simulink model "simulation_UMFCBF"  (R2022a)
settings: Solver=VariableStepAuto  StartTime=0.0  StopTime=simTime  RelTol=1e-3
values from neighbouring files (symbols this model uses):
  a = 0.20    (= 0.2)    [setup_UMFCBF.m]
  Icm = 1/2*m*robot_radius^2    (= 0.225)    [setup_UMFCBF.m]
  Kd = 100    [setup_UMFCBF.m]
  Kp = 2    [setup_UMFCBF.m]
  m = 5    [setup_UMFCBF.m]
  qg = [4 ; -1]    [setup_UMFCBF.m]
  qstart = [-2 0.1 0]'    [setup_UMFCBF.m]
  threshold_skip = 0    [setup_UMFCBF.m]
undefined symbols (not defined in the file or in its folder): clearance, obs, q0, r
libraries: slctrlblks x1
settings Model: Creator=mirkomizzoni  LastModifiedBy=dennis

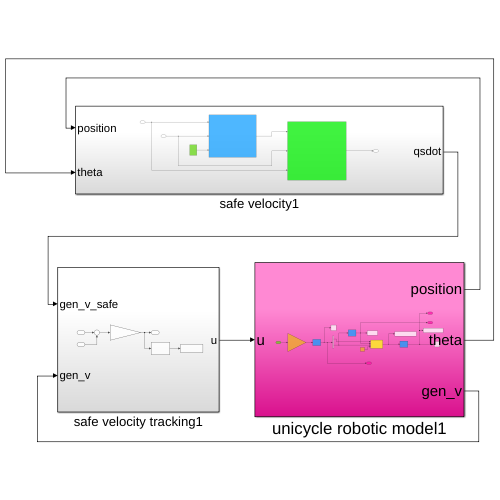
[thumbnail: Simulink's stored preview of the top-level diagram]
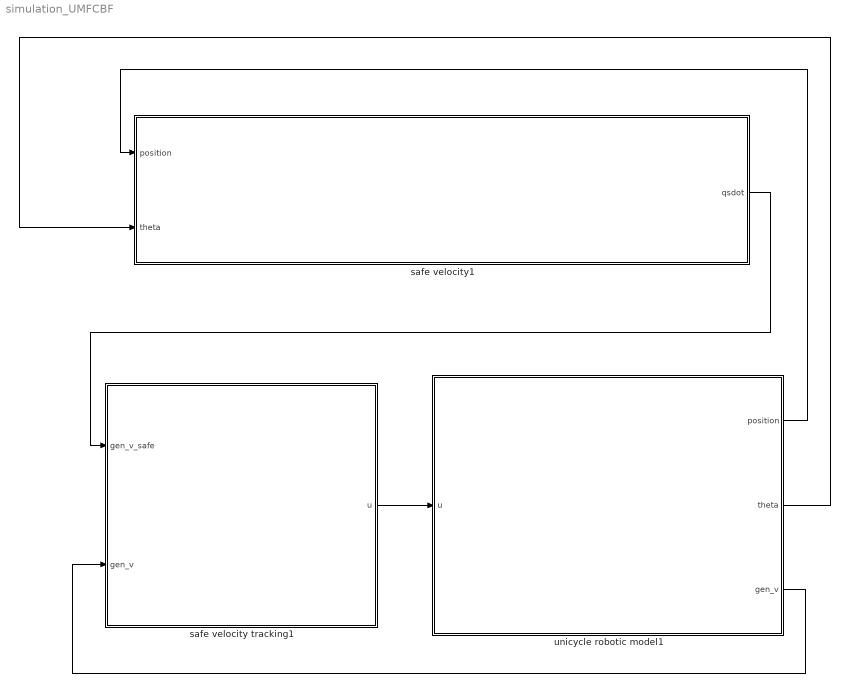
== system simulation_UMFCBF ==
  safe velocity tracking1 : Subsystem
  safe velocity1 : Subsystem
  unicycle robotic model1 : Subsystem
  wires:
  safe velocity1/1(qsdot) -> safe velocity tracking1/1(gen_v_safe)
  safe velocity tracking1/1(u) -> unicycle robotic model1/1(u)
  unicycle robotic model1/3(gen_v) -> safe velocity tracking1/2(gen_v)
  unicycle robotic model1/1(position) -> safe velocity1/1(position)
  unicycle robotic model1/2(theta) -> safe velocity1/2(theta)

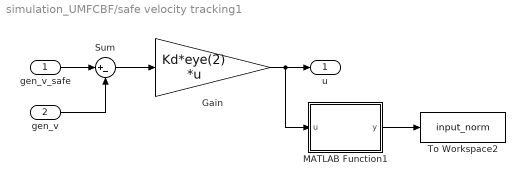
== system simulation_UMFCBF/safe velocity tracking1 ==
  gen_v_safe : Inport
  gen_v : Inport  Port=2
  Gain : Gain  Gain=Kd*eye(2)  Multiplication=Matrix(K*u)
  MATLAB Function1 : MATLAB Function  TreatAsAtomicUnit=on
  Sum : Sum  Inputs=|+-
  To Workspace2 : ToWorkspace  VariableName=input_norm  SaveFormat=Timeseries  SampleTime=0.01
  u : Outport
  wires:
  gen_v/1 -> Sum/2
  gen_v_safe/1 -> Sum/1
  Sum/1 -> Gain/1
  Gain/1 -> u/1, MATLAB Function1/1(u)
  MATLAB Function1/1(y) -> To Workspace2/1

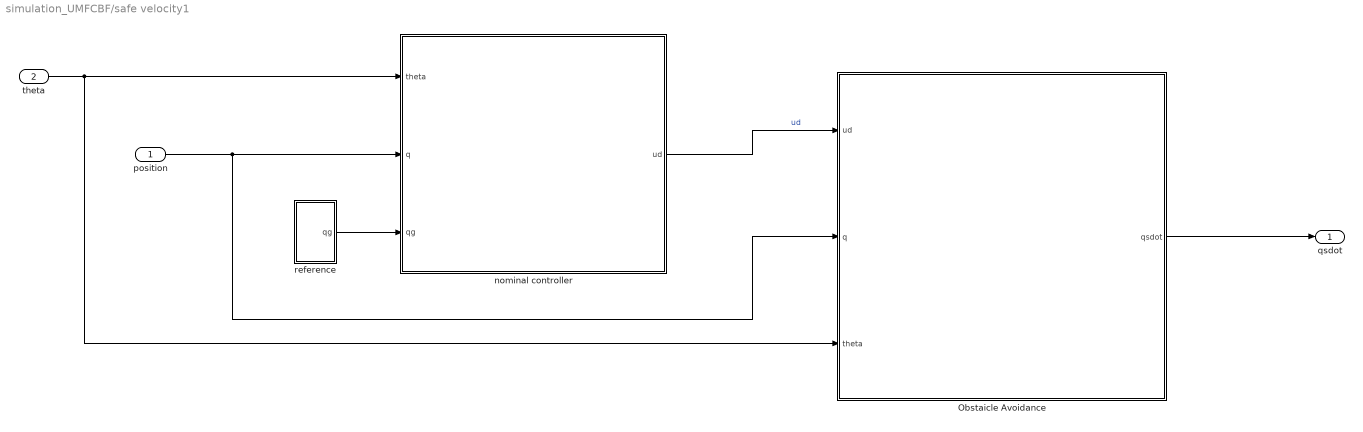
== system simulation_UMFCBF/safe velocity1 ==
  position : Inport
  theta : Inport  Port=2
  Obstaicle Avoidance : Subsystem
  nominal controller : Subsystem
  reference : Subsystem
  qsdot : Outport
  wires:
  reference/1(qg) -> nominal controller/3(qg)
  nominal controller/1(ud) -> Obstaicle Avoidance/1(ud)  "ud"
  Obstaicle Avoidance/1(qsdot) -> qsdot/1
  position/1 -> nominal controller/2(q), Obstaicle Avoidance/2(q)
  theta/1 -> Obstaicle Avoidance/3(theta), nominal controller/1(theta)

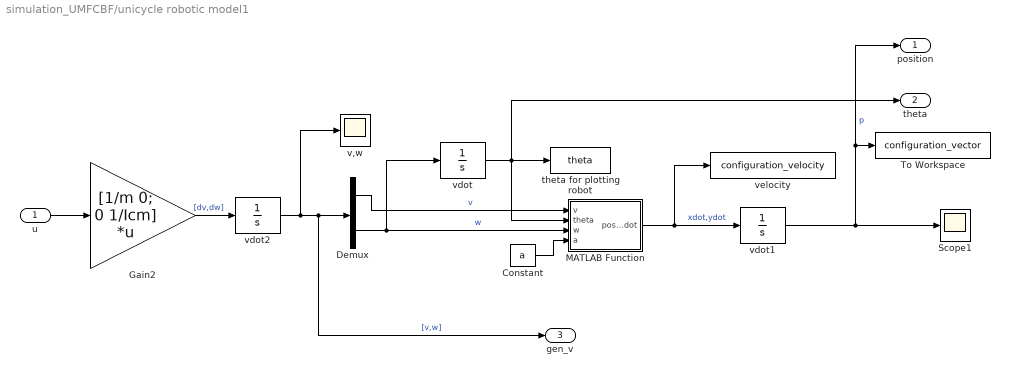
== system simulation_UMFCBF/unicycle robotic model1 ==
  u : Inport
  Constant : Constant  Value=a
  Demux : Demux  Outputs=2
  Gain2 : Gain  Gain=[1/m 0; 0 1/Icm]  Multiplication=Matrix(K*u)
  MATLAB Function : MATLAB Function  TreatAsAtomicUnit=on
  Scope1 : Scope
  To Workspace : ToWorkspace  VariableName=configuration_vector  SaveFormat=Timeseries  SampleTime=0.01
  theta for plotting robot : ToWorkspace  VariableName=theta  SaveFormat=Timeseries  SampleTime=0.01
  v,w : Scope
  vdot : Integrator  InitialCondition=q0(3)
  vdot1 : Integrator  InitialCondition=qstart
  vdot2 : Integrator  InitialCondition=[q0(4); q0(5)]
  velocity : ToWorkspace  VariableName=configuration_velocity  SaveFormat=Timeseries  SampleTime=0.01
  position : Outport
  theta : Outport  Port=2
  gen_v : Outport  Port=3
  wires:
  vdot/1 -> theta/1, theta for plotting robot/1, MATLAB Function/2(theta)
  Demux/2 -> vdot/1, MATLAB Function/3(w)  "w"
  vdot2/1 -> v,w/1, gen_v/1, Demux/1  "[v,w]"
  MATLAB Function/1(positiondot) -> velocity/1, vdot1/1  "xdot,ydot"
  Constant/1 -> MATLAB Function/4(a)
  Gain2/1 -> vdot2/1  "[dv,dw]"
  Demux/1 -> MATLAB Function/1(v)  "v"
  u/1 -> Gain2/1
  vdot1/1 -> position/1, To Workspace/1, Scope1/1  "p"

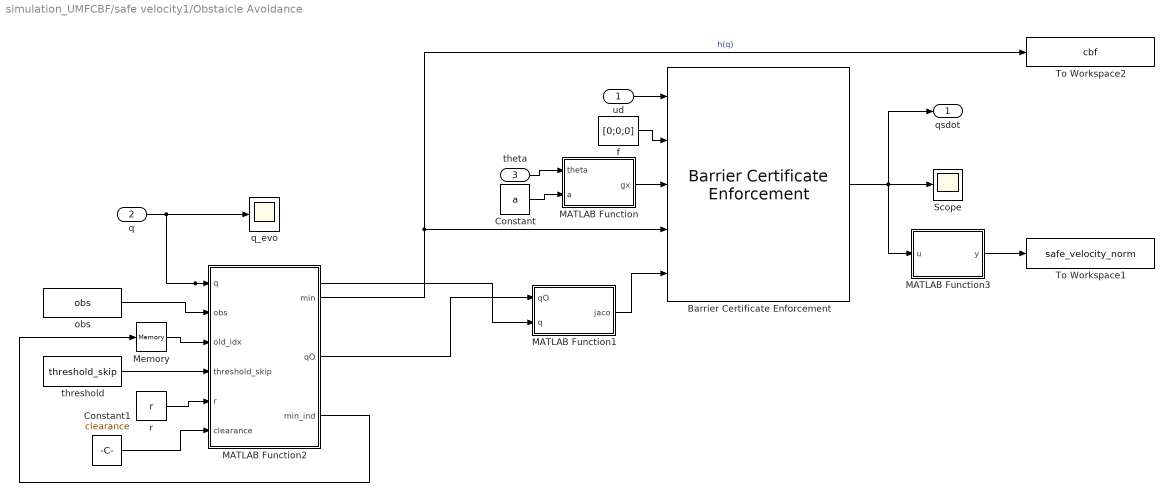
== system simulation_UMFCBF/safe velocity1/Obstaicle Avoidance ==
  ud : Inport
  q : Inport  Port=2
  theta : Inport  Port=3
  Barrier Certificate Enforcement : slctrlblks/Barrier Certificate Enforcement  nx=3  nu=2  nc=1  gamma=alpha  beta=1  external_umax=off  external_umin=off  Ts=0.01  maxiter=200  tol=1e-06  output_exitflag=off
      settings: SourceProductBaseCode=SD
  Constant : Constant  Value=a
  Constant1 : Constant  Value=clearance
  MATLAB Function : MATLAB Function  TreatAsAtomicUnit=on
  MATLAB Function1 : MATLAB Function  TreatAsAtomicUnit=on
  MATLAB Function2 : MATLAB Function  TreatAsAtomicUnit=on
  MATLAB Function3 : MATLAB Function  TreatAsAtomicUnit=on
  Memory : Memory  InitialCondition=1
  Scope : Scope
  To Workspace1 : ToWorkspace  VariableName=safe_velocity_norm  SaveFormat=Timeseries  SampleTime=0.01
  To Workspace2 : ToWorkspace  VariableName=cbf  SaveFormat=Timeseries  SampleTime=0.01
  f : Constant  Value=[0;0;0]  VectorParams1D=off
  obs : Constant  Value=obs  VectorParams1D=off
  q_evo : Scope
  r : Constant  Value=r
  threshold : Constant  Value=threshold_skip  VectorParams1D=off
  qsdot : Outport
  wires:
  MATLAB Function2/2(qO) -> MATLAB Function1/1(qO)
  q/1 -> MATLAB Function2/1(q), MATLAB Function1/2(q), q_evo/1
  MATLAB Function2/3(min_ind) -> Memory/1
  MATLAB Function3/1(y) -> To Workspace1/1
  MATLAB Function2/1(min) -> To Workspace2/1, Barrier Certificate Enforcement/4  "h(q)"
  threshold/1 -> MATLAB Function2/4(threshold_skip)
  f/1 -> Barrier Certificate Enforcement/2
  MATLAB Function1/1(jaco) -> Barrier Certificate Enforcement/5
  ud/1 -> Barrier Certificate Enforcement/1
  obs/1 -> MATLAB Function2/2(obs)
  Memory/1 -> MATLAB Function2/3(old_idx)
  Barrier Certificate Enforcement/1 -> MATLAB Function3/1(u), Scope/1, qsdot/1
  r/1 -> MATLAB Function2/5(r)
  MATLAB Function/1(gx) -> Barrier Certificate Enforcement/3
  Constant/1 -> MATLAB Function/2(a)
  theta/1 -> MATLAB Function/1(theta)
  Constant1/1 -> MATLAB Function2/6(clearance)

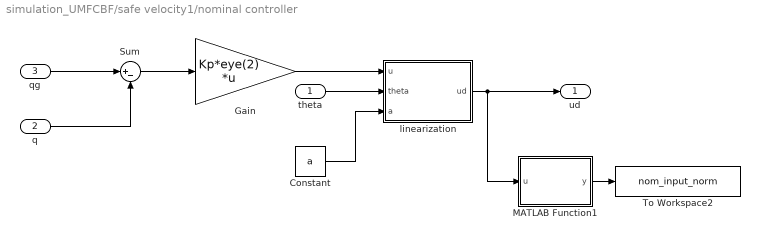
== system simulation_UMFCBF/safe velocity1/nominal controller ==
  theta : Inport
  q : Inport  Port=2
  qg : Inport  Port=3
  Constant : Constant  Value=a
  Gain : Gain  Gain=Kp*eye(2)  Multiplication=Matrix(K*u)
  MATLAB Function1 : MATLAB Function  TreatAsAtomicUnit=on
  Sum : Sum  Inputs=|+-
  To Workspace2 : ToWorkspace  VariableName=nom_input_norm  SaveFormat=Timeseries  SampleTime=0.01
  linearization : MATLAB Function  TreatAsAtomicUnit=on
  ud : Outport
  wires:
  MATLAB Function1/1(y) -> To Workspace2/1
  q/1 -> Sum/2
  qg/1 -> Sum/1
  Sum/1 -> Gain/1
  linearization/1(ud) -> ud/1, MATLAB Function1/1(u)
  Gain/1 -> linearization/1(u)
  theta/1 -> linearization/2(theta)
  Constant/1 -> linearization/3(a)

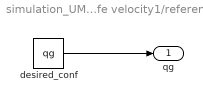
== system simulation_UMFCBF/safe velocity1/reference ==
  desired_conf : Constant  Value=qg
  qg : Outport
  wires:
  desired_conf/1 -> qg/1

== matlab function simulation_UMFCBF/safe velocity tracking1/MATLAB Function1 ==
  data: u input; y output
function y = norm_func(u)
        
y = norm(u);

== matlab function simulation_UMFCBF/safe velocity1/Obstaicle Avoidance/MATLAB Function1 ==
  data: qO input; jaco output; q input
function jaco = jacob(qO,q)
   jac = (q-qO)'/norm(q-qO);
   jaco = [jac(1) jac(2) 0];
end

== matlab function simulation_UMFCBF/safe velocity1/Obstaicle Avoidance/MATLAB Function2 ==
  data: min output; q input; obs input; qO output; min_ind output; old_idx input; threshold_skip input; r input; clearance input
function [min,qO,min_ind] = min_dist(q, obs, old_idx, threshold_skip, r, clearance)
[~,n] = size(obs);
min = norm(q-obs(:,1))-r(1);
min_ind = 1;
for i=2:n
    t = norm(q-obs(:,i))-r(i);
    if t<min
        min_ind = i;
        min = t;
    end
end

old_dist = norm(q-obs(:,old_idx))-r(old_idx);
if abs(old_dist-min) < threshold_skip
    qO = obs(:,old_idx);
    min_ind = old_idx;
    min = old_dist;
else
    qO = obs(:,min_ind);
end
min = min - clearance;
end

== matlab function simulation_UMFCBF/safe velocity1/Obstaicle Avoidance/MATLAB Function3 ==
  data: u input; y output
function y = norm_func(u)
        
y = norm(u);

== matlab function simulation_UMFCBF/safe velocity1/nominal controller/MATLAB Function1 ==
  data: u input; y output
function y = norm_func(u)
        
y = norm(u);

== matlab function simulation_UMFCBF/unicycle robotic model1/MATLAB Function ==
  data: v input; positiondot output; theta input; w input; a input
function positiondot = posdot(v,theta,w,a)
        dx = v*cos(theta)-w*a*sin(theta);
        dy = v*sin(theta)+w*a*cos(theta);
        positiondot = [dx;dy];
end

== matlab function simulation_UMFCBF/safe velocity1/nominal controller/linearization ==
  data: u input; ud output; theta input; a input
function ud = transf_T(u, theta, a)
    Tm1 = [cos(theta) sin(theta); -sin(theta)/a cos(theta)/a];
    ud = Tm1*u;
end

== matlab function simulation_UMFCBF/safe velocity1/Obstaicle Avoidance/MATLAB Function ==
  data: theta input; gx output; a input
function gx = g(theta, a)
    gx = [cos(theta) -a*sin(theta); sin(theta) a*cos(theta); 0 1];
end
